simulink model "gantrycrane_animation"  (Simulink 8.3)
settings: Solver=ode45  StartTime=0.0  StopTime=1000  RelTol=1e-3
undefined symbols (not defined in the file or in its folder): drawGantryCrane
libraries: simulink x1
settings Model: Creator=nedward  LastModifiedBy=jhl48
settings OptimizationCC: ExpressionDepthLimit=2147483647
settings DebuggingCC: FcnCallInpInsideContextMsg=UseLocalSettings

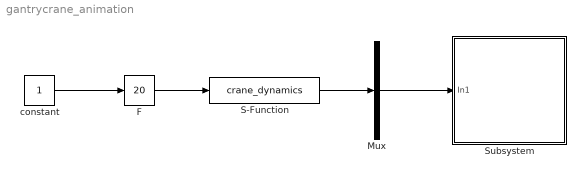
== system gantrycrane_animation ==
  F : simulink/Math Operations/Slider Gain  low=-100  gain=20  high=100
  Mux : Mux  Inputs=1
  S-Function : S-Function  FunctionName=crane_dynamics  Parameters=AP  EnableBusSupport=off
  Subsystem : Subsystem
      mask init:
      | bar = 20;
      | crane = [5 3];
      | L1 = 5;
      | R1 = 1;
      | L2 = 10;
      | R2 = 0.5;
      mask Display: image(imread('tv.jpg'))
  constant : Constant
  wires:
  constant/1 -> F/1
  Mux/1 -> Subsystem/1(In1)
  F/1 -> S-Function/1
  S-Function/1 -> Mux/1

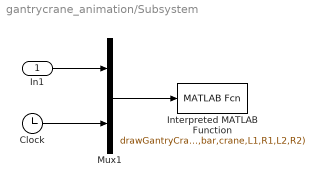
== system gantrycrane_animation/Subsystem ==
  In1 : Inport
  Clock : Clock
  Interpreted MATLAB Function : MATLABFcn  MATLABFcn=drawGantryCrane(u,bar,crane,L1,R1,L2,R2)  OutputDimensions=0  SampleTime=0.1
  Mux1 : Mux  Inputs=2
  wires:
  Clock/1 -> Mux1/2
  Mux1/1 -> Interpreted MATLAB Function/1
  In1/1 -> Mux1/1
